simulink model "FourWheelSim_base"  (R2021b)
settings: Solver=ode4  StartTime=0.0  StopTime=100  FixedStep=0.001  EnableMultiTasking=on
values from neighbouring files (symbols this model uses):
  a_f = [1.434106444513048,-3.490394354141787e-04,2.761516722659314,6.000050177239062e+04,2.990012596710455e+03,-1.736376596503330e-04,0.526021936511837]    [VehicleParams20_ver230707.m]
  a_r = a_f    [VehicleParams20_ver230707.m]
  afx_f = [1.736519934348130,-2.903281841026900e-04,2.651682004580759,7.000047010028531e+04,3.270011055825476e+03,-0.001252141095807,1.596836353939939]    [VehicleParams20_ver230707.m]
  afx_r = afx_f    [VehicleParams20_ver230707.m]
  agx_f = [0.230000000000000,2.936116597489246e+04,7.137436879966481e+03,0,0]    [VehicleParams20_ver230707.m]
  agx_r = agx_f    [VehicleParams20_ver230707.m]
  agy_f = [0.852564208514954,3.000069064154418e+04,2.070023877794581e+03,-5.089267464508360e-04,0.519364283925805]    [VehicleParams20_ver230707.m]
  agy_r = agy_f    [VehicleParams20_ver230707.m]
  b_f = [3.436650779629654,1.566044221042620e-05,0.028598122547093,3.408741969645286e+03,5.995144285148312e+03,-1.736376595720277e-04,0.526021936449385]    [VehicleParams20_ver230707.m]
  Brake_Factor = 0.66    [VehicleParams20_ver230707.m]
  Cd = Cd/(40/3.6)^2    (= 0.6885)    [VehicleParams20_ver230707.m]
  CLF = DFf/40/40    (= 0.06)    [VehicleParams20_ver230707.m]
  CLR = DFr/40/40    (= 0.065)    [VehicleParams20_ver230707.m]
  cPiston_Area_F = 2*pi*(0.0254/2)^2    (= 0.00101341495819)    [VehicleParams20_ver230707.m]
  cPiston_Area_R = 2*pi*(0.0254/2)^2    (= 0.00101341495819)    [VehicleParams20_ver230707.m]
  delta = 15.5    [VehicleParams20_ver230707.m]
  df = 1.225    [VehicleParams20_ver230707.m]
  dr = 1.225    [VehicleParams20_ver230707.m]
  eff_Radius_F = (180/2-13.5)/1000    (= 0.0765)    [VehicleParams20_ver230707.m]
  eff_Radius_R = (180/2-13.5)/1000    (= 0.0765)    [VehicleParams20_ver230707.m]
  Fd = 60*2    (= 120)    [VehicleParams20_ver230707.m]
  Frtoe = 0    [VehicleParams20_ver230707.m]
  gear_f = 13.75    [VehicleParams20_ver230707.m]
  gear_r = 13.75    [VehicleParams20_ver230707.m]
  hg = 0.28    [VehicleParams20_ver230707.m]
  HV_voltage = 600    [VehicleParams20_ver230707.m]
  I = 112    [VehicleParams20_ver230707.m]
  ini_v = ini_speed/3.6    (= 10.4166666667)    [VehicleParams20_ver230707.m]
  Kframe = 5.94*10^6    (= 5940000)    [VehicleParams20_ver230707.m]
  kk_f = 2800*180/pi    (= 160428.182637)    [VehicleParams20_ver230707.m]
  kk_r = 4200*180/pi    (= 240642.273955)    [VehicleParams20_ver230707.m]
  krfr = 0.5    [VehicleParams20_ver230707.m]
  l = 1.530    (= 1.53)    [VehicleParams20_ver230707.m]
  lf = l*(1-WBf)    (= 0.7956)    [VehicleParams20_ver230707.m]
  lr = l*WBf    (= 0.7344)    [VehicleParams20_ver230707.m]
  M = 200+60    (= 260)    [VehicleParams20_ver230707.m]
  mu_tire_F = 0.587-0.587+0.55    (= 0.55)    [VehicleParams20_ver230707.m]
  mu_tire_R = 0.587-0.587+0.55    (= 0.55)    [VehicleParams20_ver230707.m]
  Mwf = Iwf/Rwf/Rwf    (= 3.82716814816)    [VehicleParams20_ver230707.m]
  Mwr = Iwr/Rwr/Rwr    (= 3.82716814816)    [VehicleParams20_ver230707.m]
  rcf = 0.000    (= 0)    [VehicleParams20_ver230707.m]
  rch = rcf*WBf+rcr*(1-WBf)    (= 0)    [VehicleParams20_ver230707.m]
  rcr = 0.000    (= 0)    [VehicleParams20_ver230707.m]
  Reartoe = -2    [VehicleParams20_ver230707.m]
  Rr_toe = Reartoe*pi/180    (= -0.0349065850399)    [VehicleParams20_ver230707.m]
  Rwf = 18*(25.4/1000)/2    (= 0.2286)    [VehicleParams20_ver230707.m]
  Rwr = 18*(25.4/1000)/2    (= 0.2286)    [VehicleParams20_ver230707.m]
  T_TireF = TireL_f/V    (= 0.036760000032)    [VehicleParams20_ver230707.m]
  T_TireR = TireL_r/V    (= 0.036760000032)    [VehicleParams20_ver230707.m]
  tspeed = 37.5    [VehicleParams20_ver230707.m]
  WBf = 0.48    [VehicleParams20_ver230707.m]
  zc_f = castrail_Fr/1000    (= 0)    [VehicleParams20_ver230707.m]
  zc_r = castrail_Rr/1000    (= 0)    [VehicleParams20_ver230707.m]
libraries: simulink x25, dspstat3 x1
(part 2 of 4)

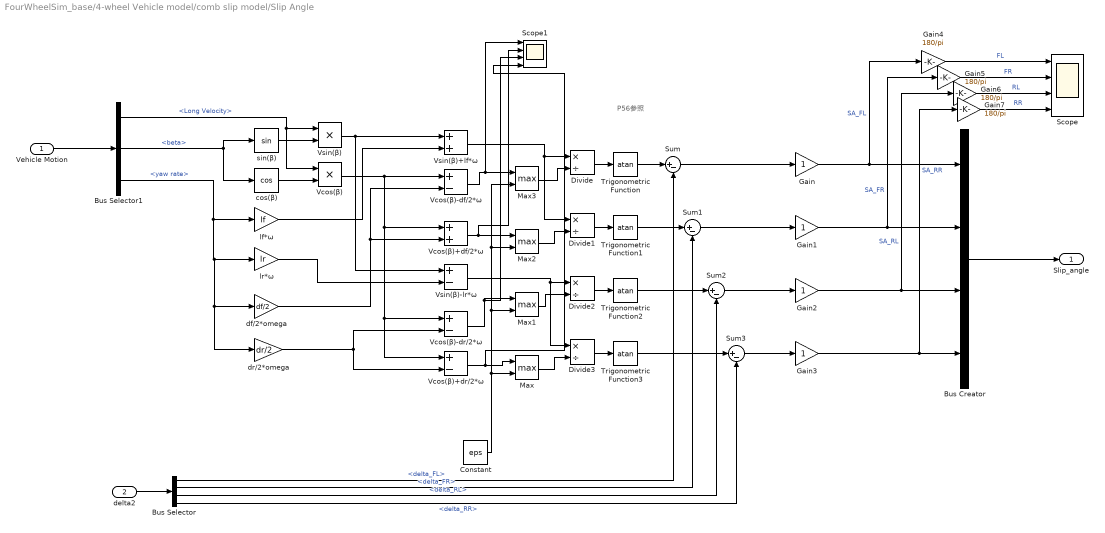
== system FourWheelSim_base/4-wheel Vehicle model/comb slip model/Slip Angle ==
  note: P56参照
  Vehicle Motion : Inport
  delta2 : Inport  Port=2
  Bus Creator : BusCreator  Inputs=4
  Bus Selector : BusSelector  OutputSignals=delta_FL,delta_FR,delta_RL,delta_RR
  Bus Selector1 : BusSelector  OutputSignals=Long Velocity,beta,yaw rate
  Constant : Constant  Value=eps
  Divide{,1..3} (4 alike) : Product  Inputs=*/
  Gain{,1..3} (4 alike) : Gain
  Gain{4..7} (4 alike) : Gain  Gain=180/pi
  Max{,1..3} (4 alike) : MinMax  Function=max  Inputs=2
  Scope : Scope  NumInputPorts=4
  Scope1 : Scope  NumInputPorts=4
  Sum{,1..3} (4 alike) : Sum  Inputs=|+-
  Trigonometric Function{,1..3} (4 alike) : Trigonometry  Operator=atan
  Vcos(β) : Product  Inputs=**
  Vcos(β)+df/2*ω : Sum
  Vcos(β)+dr/2*ω : Sum  Inputs=+-
  Vcos(β)-df/2*ω : Sum  Inputs=+-
  Vcos(β)-dr/2*ω : Sum  Inputs=+-
  Vsin(β) : Product  Inputs=**
  Vsin(β)+lf*ω : Sum
  Vsin(β)-lr*ω : Sum  Inputs=+-
  cos(β) : Trigonometry  Operator=cos
  df/2*omega : Gain  Gain=df/2
  dr/2*omega : Gain  Gain=dr/2
  lf*ω : Gain  Gain=lf
  lr*ω : Gain  Gain=lr
  sin(β) : Trigonometry
  Slip_angle : Outport  VectorParamsAs1DForOutWhenUnconnected=off
  wires:
  Bus Selector1/2 -> sin(β)/1, cos(β)/1  "<beta>"
  Bus Selector1/3 -> dr/2*omega/1, df/2*omega/1, lr*ω/1, lf*ω/1  "<yaw rate>"
  sin(β)/1 -> Vsin(β)/2
  cos(β)/1 -> Vcos(β)/2
  Vsin(β)/1 -> Vsin(β)-lr*ω/1, Vsin(β)+lf*ω/1
  lf*ω/1 -> Vsin(β)+lf*ω/2
  df/2*omega/1 -> Vcos(β)+df/2*ω/2, Vcos(β)-df/2*ω/2
  Vsin(β)+lf*ω/1 -> Divide1/1, Divide/1
  lr*ω/1 -> Vsin(β)-lr*ω/2
  Vcos(β)/1 -> Vcos(β)+df/2*ω/1, Vcos(β)+dr/2*ω/1, Vcos(β)-dr/2*ω/1, Vcos(β)-df/2*ω/1
  dr/2*omega/1 -> Vcos(β)-dr/2*ω/2, Vcos(β)+dr/2*ω/2
  Vsin(β)-lr*ω/1 -> Divide3/1, Divide2/1
  Bus Selector/1 -> Sum/2  "<delta_FL>"
  Trigonometric Function/1 -> Sum/1
  Sum/1 -> Gain/1
  Bus Selector/2 -> Sum1/2  "<delta_FR>"
  Trigonometric Function1/1 -> Sum1/1
  Sum1/1 -> Gain1/1
  Bus Selector/3 -> Sum2/2  "<delta_RL>"
  Trigonometric Function2/1 -> Sum2/1
  Bus Selector/4 -> Sum3/2  "<delta_RR>"
  Trigonometric Function3/1 -> Sum3/1
  Sum3/1 -> Gain3/1
  Sum2/1 -> Gain2/1
  Gain/1 -> Gain4/1, Bus Creator/1  "SA_FL"
  Gain1/1 -> Gain5/1, Bus Creator/2  "SA_FR"
  Gain2/1 -> Bus Creator/3, Gain6/1  "SA_RL"
  Gain3/1 -> Gain7/1, Bus Creator/4  "SA_RR"
  Bus Selector1/1 -> Vsin(β)/1, Vcos(β)/1  "<Long Velocity>"
  Bus Creator/1 -> Slip_angle/1
  delta2/1 -> Bus Selector/1
  Vehicle Motion/1 -> Bus Selector1/1
  Divide3/1 -> Trigonometric Function3/1
  Divide2/1 -> Trigonometric Function2/1
  Divide1/1 -> Trigonometric Function1/1
  Divide/1 -> Trigonometric Function/1
  Constant/1 -> Max3/2, Max2/2, Max1/2, Max/2
  Vcos(β)+dr/2*ω/1 -> Scope1/4, Max/1
  Vcos(β)+df/2*ω/1 -> Scope1/2, Max2/1
  Vcos(β)-df/2*ω/1 -> Scope1/1, Max3/1
  Vcos(β)-dr/2*ω/1 -> Scope1/3, Max1/1
  Max3/1 -> Divide/2
  Max2/1 -> Divide1/2
  Max1/1 -> Divide2/2
  Max/1 -> Divide3/2
  Gain4/1 -> Scope/1  "FL"
  Gain5/1 -> Scope/2  "FR"
  Gain6/1 -> Scope/3  "RL"
  Gain7/1 -> Scope/4  "RR"

== system FourWheelSim_base/4-wheel Vehicle model/comb slip model/Slip rate calc ==
  VehicleSpeed : Inport
  Wheel Speed : Inport  Port=2
  Bus Creator : BusCreator  Inputs=4
  Bus Selector : BusSelector  OutputSignals=Wheel_Speed_FL,Wheel_Speed_FR,Wheel_Speed_RL,Wheel_Speed_RR
  Bus Selector1 : BusSelector  OutputSignals=Long Velocity
  SlipRateClc{,1..3} (4 alike) : Subsystem  ReferencedSubsystem=SlipRateClc
  "SlipRate " : Outport  VectorParamsAs1DForOutWhenUnconnected=off
  wires:
  SlipRateClc2/1 -> Bus Creator/3  "Sliprate_RL"
  SlipRateClc1/1 -> Bus Creator/2  "Sliprate_FR"
  SlipRateClc/1 -> Bus Creator/1  "Sliprate_FL"
  SlipRateClc3/1 -> Bus Creator/4  "Sliprate_RR"
  Bus Selector1/1 -> SlipRateClc3/2, SlipRateClc2/2, SlipRateClc1/2, SlipRateClc/2  "<Long Velocity>"
  Bus Creator/1 -> "SlipRate "/1
  Wheel Speed/1 -> Bus Selector/1
  Bus Selector/4 -> SlipRateClc3/1  "<Wheel_Speed_RR>"
  Bus Selector/2 -> SlipRateClc1/1  "<Wheel_Speed_FR>"
  Bus Selector/1 -> SlipRateClc/1  "<Wheel_Speed_FL>"
  VehicleSpeed/1 -> Bus Selector1/1
  Bus Selector/3 -> SlipRateClc2/1  "<Wheel_Speed_RL>"

== system FourWheelSim_base/4-wheel Vehicle model/comb slip model/Wheel speed calc ==
  note: Unit : m/s
  comb_Fx : Inport
  Torque : Inport  Port=2
  1/r : Gain  Gain=1/Rwf
  1/r1 : Gain  Gain=1/Rwf
  1/r2 : Gain  Gain=1/Rwr
  1/r3 : Gain  Gain=1/Rwr
  Bus Creator : BusCreator  Inputs=4
  Bus Selector : BusSelector  OutputSignals=FL,RL,FR,RR
  Bus Selector1 : BusSelector  OutputSignals=Fx.Fx_FL,Fx.Fx_RL,Fx.Fx_FR,Fx.Fx_RR
  Gain17 : Gain  Gain=1/Mwf
  Gain18 : Gain  Gain=1/Mwf
  Gain19 : Gain  Gain=1/Mwr
  Gain20 : Gain  Gain=1/Mwr
  Scope : Scope  NumInputPorts=4
  Scope1 : Scope  NumInputPorts=4
  Scope2 : Scope  NumInputPorts=4
  Sum{2..3,13..14} (4 alike) : Sum  Inputs=|+-
  wheel speed F_in : Integrator  InitialCondition=ini_v  LimitOutput=on  LowerSaturationLimit=0
  wheel speed F_out : Integrator  InitialCondition=ini_v  LimitOutput=on  LowerSaturationLimit=0
  wheel speed R_in : Integrator  InitialCondition=ini_v  LimitOutput=on  LowerSaturationLimit=0
  wheel speed R_out : Integrator  InitialCondition=ini_v  LimitOutput=on  LowerSaturationLimit=0
  Wheel Speed : Outport  VectorParamsAs1DForOutWhenUnconnected=off
  wires:
  wheel speed R_out/1 -> Scope/4, Bus Creator/4  "Wheel_Speed_RR"
  Sum2/1 -> Gain18/1
  Sum14/1 -> Gain19/1
  wheel speed F_in/1 -> Scope/1, Bus Creator/1  "Wheel_Speed_FL"
  Gain19/1 -> wheel speed R_in/1
  Gain18/1 -> wheel speed F_out/1
  Sum3/1 -> Gain17/1
  Gain17/1 -> wheel speed F_in/1
  Sum13/1 -> Gain20/1
  Gain20/1 -> wheel speed R_out/1
  wheel speed F_out/1 -> Scope/2, Bus Creator/2  "Wheel_Speed_RL"
  wheel speed R_in/1 -> Scope/3, Bus Creator/3  "Wheel_Speed_FR"
  Bus Creator/1 -> Wheel Speed/1
  Torque/1 -> Bus Selector/1
  Bus Selector/1 -> Scope1/1, 1/r/1  "<FL>"
  Bus Selector/2 -> Scope1/2, 1/r2/1  "<RL>"
  Bus Selector/3 -> Scope1/3, 1/r1/1  "<FR>"
  Bus Selector/4 -> 1/r3/1, Scope1/4  "<RR>"
  comb_Fx/1 -> Bus Selector1/1
  Bus Selector1/1 -> Scope2/1, Sum3/2  "<Fx_FL>"
  Bus Selector1/2 -> Scope2/2, Sum2/2  "<Fx_RL>"
  Bus Selector1/3 -> Scope2/3, Sum14/2  "<Fx_FR>"
  Bus Selector1/4 -> Scope2/4, Sum13/2  "<Fx_RR>"
  1/r/1 -> Sum3/1
  1/r1/1 -> Sum14/1
  1/r2/1 -> Sum2/1
  1/r3/1 -> Sum13/1

== system FourWheelSim_base/4-wheel Vehicle model/comb slip model/comb Fx calc ==
  tire status : Inport
  Bus Creator : BusCreator  Inputs=4
  Bus Selector : BusSelector  OutputSignals=load.Load_FL,Slip angle.SA_FL,Slip rate.Sliprate_FL
  Bus Selector1 : BusSelector  OutputSignals=load.Load_FR,Slip angle.SA_FR,Slip rate.Sliprate_FR
  Bus Selector2 : BusSelector  OutputSignals=load.Load_RL,Slip angle.SA_RL,Slip rate.Sliprate_RL
  Bus Selector3 : BusSelector  OutputSignals=load.Load_RR,Slip angle.SA_RR,Slip rate.Sliprate_RR
  Force_Fin_comb_FX : Subsystem
  Force_Fout_comb_FX : Subsystem
  Force_Rin_comb_FX : Subsystem
  Force_Rout_comb1_FX : Subsystem
  Fx : Outport  VectorParamsAs1DForOutWhenUnconnected=off
  wires:
  Bus Creator/1 -> Fx/1
  Force_Fout_comb_FX/1(Force_Fout) -> Bus Creator/2  "Fx_FR"
  Force_Fin_comb_FX/1(Force_Fin) -> Bus Creator/1  "Fx_FL"
  Force_Rin_comb_FX/1(Force_Rin) -> Bus Creator/3  "Fx_RL"
  Force_Rout_comb1_FX/1(Force_Rin) -> Bus Creator/4  "Fx_RR"
  tire status/1 -> Bus Selector3/1, Bus Selector2/1, Bus Selector/1, Bus Selector1/1
  Bus Selector/1 -> Force_Fin_comb_FX/1(W_Fin)  "<Load_FL>"
  Bus Selector/2 -> Force_Fin_comb_FX/2(beta_Fin)  "<SA_FL>"
  Bus Selector/3 -> Force_Fin_comb_FX/3(slip rate)  "<Sliprate_FL>"
  Bus Selector1/1 -> Force_Fout_comb_FX/1(W_Fout)  "<Load_FR>"
  Bus Selector1/2 -> Force_Fout_comb_FX/2(beta_Fout)  "<SA_FR>"
  Bus Selector1/3 -> Force_Fout_comb_FX/3(slip rate)  "<Sliprate_FR>"
  Bus Selector2/1 -> Force_Rin_comb_FX/1(W_Rin)  "<Load_RL>"
  Bus Selector2/2 -> Force_Rin_comb_FX/2(beta_Rin)  "<SA_RL>"
  Bus Selector2/3 -> Force_Rin_comb_FX/3(slip rate)  "<Sliprate_RL>"
  Bus Selector3/1 -> Force_Rout_comb1_FX/1(W_Rout)  "<Load_RR>"
  Bus Selector3/2 -> Force_Rout_comb1_FX/2(beta_Rout)  "<SA_RR>"
  Bus Selector3/3 -> Force_Rout_comb1_FX/3(slip rate)  "<Sliprate_RR>"

== system FourWheelSim_base/4-wheel Vehicle model/comb slip model/comb Fy calc ==
  tire status : Inport
  Bus Creator : BusCreator  Inputs=4
  Bus Selector : BusSelector  OutputSignals=load.Load_FL,Slip angle.SA_FL,Slip rate.Sliprate_FL
  Bus Selector1 : BusSelector  OutputSignals=load.Load_FR,Slip angle.SA_FR,Slip rate.Sliprate_FR
  Bus Selector2 : BusSelector  OutputSignals=load.Load_RL,Slip angle.SA_RL,Slip rate.Sliprate_RL
  Bus Selector3 : BusSelector  OutputSignals=load.Load_RR,Slip angle.SA_RR,Slip rate.Sliprate_RR
  Force_Fin_comb_FY : Subsystem
  Force_Fout_comb_FY : Subsystem
  Force_Rin_comb_FY : Subsystem
  Force_Rout_comb_FY : Subsystem
  Fy : Outport  VectorParamsAs1DForOutWhenUnconnected=off
  wires:
  Bus Creator/1 -> Fy/1
  Force_Fout_comb_FY/1(Force_Fout) -> Bus Creator/2  "Fy_FR"
  Force_Fin_comb_FY/1(Force_Fin) -> Bus Creator/1  "Fy_FL"
  Force_Rin_comb_FY/1(Force_Rin) -> Bus Creator/3  "Fy_RL"
  Force_Rout_comb_FY/1(Force_Rout) -> Bus Creator/4  "Fy_RR"
  Bus Selector/3 -> Force_Fin_comb_FY/3(slip rate)  "<Sliprate_FL>"
  Bus Selector3/3 -> Force_Rout_comb_FY/3(slip rate)  "<Sliprate_RR>"
  Bus Selector2/1 -> Force_Rin_comb_FY/1(W_Fin)  "<Load_RL>"
  Bus Selector1/1 -> Force_Fout_comb_FY/1(W_Fin)  "<Load_FR>"
  Bus Selector1/2 -> Force_Fout_comb_FY/2(beta_Fin)  "<SA_FR>"
  tire status/1 -> Bus Selector3/1, Bus Selector2/1, Bus Selector/1, Bus Selector1/1
  Bus Selector1/3 -> Force_Fout_comb_FY/3(slip rate)  "<Sliprate_FR>"
  Bus Selector2/3 -> Force_Rin_comb_FY/3(slip rate)  "<Sliprate_RL>"
  Bus Selector2/2 -> Force_Rin_comb_FY/2(beta_Fin)  "<SA_RL>"
  Bus Selector/2 -> Force_Fin_comb_FY/2(beta_Fin)  "<SA_FL>"
  Bus Selector/1 -> Force_Fin_comb_FY/1(W_Fin)  "<Load_FL>"
  Bus Selector3/2 -> Force_Rout_comb_FY/2(beta_Fin)  "<SA_RR>"
  Bus Selector3/1 -> Force_Rout_comb_FY/1(W_Fin)  "<Load_RR>"

== system FourWheelSim_base/4-wheel Vehicle model/equation of motion /Beta Angle ==
  Lat Velo : Inport
  Long Velo : Inport  Port=2
  Atan : Trigonometry  Operator=atan
  Constant : Constant  Value=eps
  Divide : Product  Inputs=*/
  Max : MinMax  Function=max  Inputs=2
  Body Beta Angle : Outport  VectorParamsAs1DForOutWhenUnconnected=off
  tag scope: B=global
  wires:
  Lat Velo/1 -> Divide/1
  Max/1 -> Divide/2
  Divide/1 -> Atan/1
  Atan/1 -> [B], Body Beta Angle/1
  Long Velo/1 -> Max/1
  Constant/1 -> Max/2

== system FourWheelSim_base/4-wheel Vehicle model/equation of motion /GPS cordinate Clc ==
  Long Velo : Inport
  Lat Velo : Inport  Port=2
  YawAngle : Inport  Port=3
  Add : Sum  Inputs=+-
  Add1 : Sum
  Cos : Trigonometry  Operator=cos
  Cos1 : Trigonometry  Operator=cos
  Divide{,1..3} (4 alike) : Product  Inputs=**
  Integrator1 : Integrator
  Integrator2 : Integrator
  Sin : Trigonometry
  Sin1 : Trigonometry
  GPS East : Outport  VectorParamsAs1DForOutWhenUnconnected=off
  GPS North : Outport  Port=2  VectorParamsAs1DForOutWhenUnconnected=off
  wires:
  Long Velo/1 -> Divide1/1, Divide/1
  Divide/1 -> Add/1
  Add1/1 -> Integrator2/1
  Cos/1 -> Divide/2
  Integrator1/1 -> GPS East/1  "GPS East"
  Sin/1 -> Divide1/2
  Integrator2/1 -> GPS North/1  "GPS North"
  Sin1/1 -> Divide3/2
  Cos1/1 -> Divide2/2
  YawAngle/1 -> Cos/1, Cos1/1, Sin/1, Sin1/1
  Lat Velo/1 -> Divide3/1, Divide2/1
  Divide3/1 -> Add/2
  Add/1 -> Integrator1/1
  Divide1/1 -> Add1/1
  Divide2/1 -> Add1/2

== system FourWheelSim_base/4-wheel Vehicle model/equation of motion /Net Long Force ==
  Vehicle speed : Inport
  Long Force : Inport  Port=2
  Delay : Delay  DelayLength=1
  Gain16 : Gain  Gain=Cd
  Product : Product
  Rolling resistance : Constant  Value=Fd
  Sum1 : Sum  Inputs=|+-
  Sum3 : Sum  Inputs=|+-
  Net Long Force : Outport  VectorParamsAs1DForOutWhenUnconnected=off
  wires:
  Sum3/1 -> Sum1/1
  Long Force/1 -> Sum3/1
  Product/1 -> Gain16/1
  Rolling resistance/1 -> Sum3/2
  Gain16/1 -> Sum1/2  "Drag Force"
  Vehicle speed/1 -> Delay/1
  Sum1/1 -> Net Long Force/1
  Delay/1 -> Product/2, Product/1

== system FourWheelSim_base/4-wheel Vehicle model/equation of motion /Roll Clc ==
  note: ロール剛性を適当に0.0001にしてあるが
      | 本来の値が求められるなら変えたい
  Lat Acc : Inport
  Add : Sum  Inputs=+-
  Constant : Constant  Value=0.001
  Delay : Delay  DelayLength=1
  Divide : Product  Inputs=*/
  Gain : Gain  Gain=180/pi
  Roll rad : Gain  Gain=M*(hg-rch)*0.0001
  Scope : Scope
  RollRate : Outport  VectorParamsAs1DForOutWhenUnconnected=off
  RollAngle : Outport  Port=2  VectorParamsAs1DForOutWhenUnconnected=off
  wires:
  Delay/1 -> Add/2
  Constant/1 -> Divide/2
  Add/1 -> Divide/1
  Lat Acc/1 -> Roll rad/1
  Roll rad/1 -> Gain/1, RollAngle/1, Delay/1, Add/1  "RollAngle"
  Divide/1 -> RollRate/1  "RollRate"
  Gain/1 -> Scope/1

== system FourWheelSim_base/4-wheel Vehicle model/equation of motion /Yaw Clc ==
  Yaw Moment : Inport
  Moment/I : Gain  Gain=1/I
  yaw angle[rad] : Integrator
  yaw rate[rad/s] : Integrator
  yaw rate : Outport  VectorParamsAs1DForOutWhenUnconnected=off
  yaw angle : Outport  Port=2  VectorParamsAs1DForOutWhenUnconnected=off
  wires:
  yaw angle[rad]/1 -> yaw angle/1  "yaw angle"
  Moment/I/1 -> yaw rate[rad/s]/1
  yaw rate[rad/s]/1 -> yaw rate/1, yaw angle[rad]/1  "yaw rate"
  Yaw Moment/1 -> Moment/I/1

== system FourWheelSim_base/4-wheel Vehicle model/equation of motion /equation of motion ==
  Net Long Force : Inport
  Lat Force : Inport  Port=2
  yaw rate : Inport  Port=3
  Add : Sum
  Add1 : Sum  Inputs=-+
  Divide : Product  Inputs=**
  Divide1 : Product  Inputs=**
  Gain2 : Gain  Gain=1/3.6
  Integrator : Integrator  InitialConditionSource=external
  Integrator1 : Integrator
  Mass : Gain  Gain=1/M
  Mass2 : Gain  Gain=1/M
  Scope : Scope  NumInputPorts=2
  Scope1 : Scope  NumInputPorts=2
  Long Acc : Outport  VectorParamsAs1DForOutWhenUnconnected=off
  Long Velo : Outport  Port=2  VectorParamsAs1DForOutWhenUnconnected=off
  Lat Acc : Outport  Port=3  VectorParamsAs1DForOutWhenUnconnected=off
  Lat Velo : Outport  Port=4  VectorParamsAs1DForOutWhenUnconnected=off
  wires:
  Divide/1 -> Add/2  "vr"
  Add/1 -> Integrator/1
  Add1/1 -> Scope1/1, Integrator1/1
  Mass2/1 -> Add/1, Long Acc/1  "Fx/M"
  Divide1/1 -> Add1/1  "ur"
  Lat Force/1 -> Mass/1
  Net Long Force/1 -> Mass2/1
  Mass/1 -> Add1/2, Scope1/2, Lat Acc/1  "Fy/M"
  Integrator1/1 -> Divide/2, Scope/2, Lat Velo/1  "v"
  Integrator/1 -> Long Velo/1, Divide1/1, Scope/1  "u"
  yaw rate/1 -> Divide1/2, Divide/1
  [TargetSpeed] -> Gain2/1
  Gain2/1 -> Integrator/2

== system FourWheelSim_base/4-wheel Vehicle model/force direction change/Lat Force and Yaw Moment1 ==
  In1 : Inport
  Bus Selector : BusSelector  OutputSignals=Fx.Fx_FL,delta sincos.sin(deltaFL)
  Bus Selector1 : BusSelector  OutputSignals=Fy.Fy_FL,delta sincos.cos(deltaFL)
  Bus Selector2 : BusSelector  OutputSignals=Fx.Fx_FR,delta sincos.sin(deltaFR)
  Bus Selector3 : BusSelector  OutputSignals=Fy.Fy_FR,delta sincos.cos(deltaFR)
  Bus Selector4 : BusSelector  OutputSignals=Fx.Fx_RL,delta sincos.sin(deltaRL)
  Bus Selector5 : BusSelector  OutputSignals=Fy.Fy_RL,delta sincos.cos(deltaRL)
  Bus Selector6 : BusSelector  OutputSignals=Fx.Fx_RR,delta sincos.sin(deltaRR)
  Bus Selector7 : BusSelector  OutputSignals=Fy.Fy_RR,delta sincos.cos(deltaRR)
  FXsin(-Rr_Toe) : Product  Inputs=**
  FXsin(Rr_Toe) : Product  Inputs=**
  FXsin(delta) : Product  Inputs=**
  FXsin(delta)1 : Product  Inputs=**
  FYcos(-Rr_Toe) : Product  Inputs=**
  FYcos(Rr_Toe) : Product  Inputs=**
  FYcos(delta) : Product  Inputs=**
  FYcos(delta)1 : Product  Inputs=**
  Lat Force : Sum  Inputs=++++
  Sum{21..24} (4 alike) : Sum  Inputs=++|
  Yaw Moment : Sum  Inputs=++++
  lf : Gain  Gain=lf
  lf1 : Gain  Gain=lf
  lr : Gain  Gain=-lr
  lr1 : Gain  Gain=-lr
  Yaw_Moment : Outport  VectorParamsAs1DForOutWhenUnconnected=off
  Lat_Force : Outport  Port=2  VectorParamsAs1DForOutWhenUnconnected=off
  wires:
  Lat Force/1 -> Lat_Force/1
  Yaw Moment/1 -> Yaw_Moment/1
  FYcos(delta)/1 -> Sum21/2
  FYcos(Rr_Toe)/1 -> Sum24/2
  Sum23/1 -> Lat Force/3, lr/1
  FXsin(delta)/1 -> Sum21/1
  FXsin(-Rr_Toe)/1 -> Sum23/1
  Sum21/1 -> Lat Force/1, lf/1
  FXsin(delta)1/1 -> Sum22/1
  FYcos(delta)1/1 -> Sum22/2
  Sum22/1 -> Lat Force/2, lf1/1
  Sum24/1 -> Lat Force/4, lr1/1
  FYcos(-Rr_Toe)/1 -> Sum23/2
  FXsin(Rr_Toe)/1 -> Sum24/1
  lf/1 -> Yaw Moment/4
  lf1/1 -> Yaw Moment/3
  lr/1 -> Yaw Moment/2
  lr1/1 -> Yaw Moment/1
  In1/1 -> Bus Selector7/1, Bus Selector6/1, Bus Selector5/1, Bus Selector4/1, Bus Selector3/1, Bus Selector2/1, Bus Selector1/1, Bus Selector/1
  Bus Selector/1 -> FXsin(delta)/1  "<Fx_FL>"
  Bus Selector/2 -> FXsin(delta)/2  "<sin(deltaFL)>"
  Bus Selector1/1 -> FYcos(delta)/1  "<Fy_FL>"
  Bus Selector1/2 -> FYcos(delta)/2  "<cos(deltaFL)>"
  Bus Selector2/1 -> FXsin(delta)1/1  "<Fx_FR>"
  Bus Selector2/2 -> FXsin(delta)1/2  "<sin(deltaFR)>"
  Bus Selector3/1 -> FYcos(delta)1/1  "<Fy_FR>"
  Bus Selector3/2 -> FYcos(delta)1/2  "<cos(deltaFR)>"
  Bus Selector4/1 -> FXsin(-Rr_Toe)/1  "<Fx_RL>"
  Bus Selector4/2 -> FXsin(-Rr_Toe)/2  "<sin(deltaRL)>"
  Bus Selector5/1 -> FYcos(-Rr_Toe)/1  "<Fy_RL>"
  Bus Selector5/2 -> FYcos(-Rr_Toe)/2  "<cos(deltaRL)>"
  Bus Selector6/1 -> FXsin(Rr_Toe)/1  "<Fx_RR>"
  Bus Selector6/2 -> FXsin(Rr_Toe)/2  "<sin(deltaRR)>"
  Bus Selector7/1 -> FYcos(Rr_Toe)/1  "<Fy_RR>"
  Bus Selector7/2 -> FYcos(Rr_Toe)/2  "<cos(deltaRR)>"

== system FourWheelSim_base/4-wheel Vehicle model/force direction change/Long Force and Vectoring Yaw Moment ==
  In1 : Inport
  Bus Selector : BusSelector  OutputSignals=Fx.Fx_FL,delta sincos.cos(deltaFL)
  Bus Selector1 : BusSelector  OutputSignals=Fy.Fy_FL,delta sincos.sin(deltaFL)
  Bus Selector2 : BusSelector  OutputSignals=Fx.Fx_FR,delta sincos.cos(deltaFR)
  Bus Selector3 : BusSelector  OutputSignals=Fy.Fy_FR,delta sincos.sin(deltaFR)
  Bus Selector4 : BusSelector  OutputSignals=Fx.Fx_RL,delta sincos.cos(deltaRL)
  Bus Selector5 : BusSelector  OutputSignals=Fy.Fy_RL,delta sincos.sin(deltaRL)
  Bus Selector6 : BusSelector  OutputSignals=Fx.Fx_RR,delta sincos.cos(deltaRL)
  Bus Selector7 : BusSelector  OutputSignals=Fy.Fy_RR,delta sincos.sin(deltaRR)
  FXcos(-Rr_Toe) : Product  Inputs=**
  "FXcos(Rr_Toe)1 " : Product  Inputs=**
  FXcos(delta) : Product  Inputs=**
  FXcos(delta)1 : Product  Inputs=**
  FYsin(-Rr_Toe) : Product  Inputs=**
  FYsin(Rr_Toe)1 : Product  Inputs=**
  FYsin(delta) : Product  Inputs=**
  FYsin(delta)1 : Product  Inputs=**
  Long Force : Sum  Inputs=++++
  Sum{17..20} (4 alike) : Sum  Inputs=|+-
  Vectoring Yaw Moment : Sum  Inputs=++++
  df/2 : Gain  Gain=-df/2
  df/2_1 : Gain  Gain=-dr/2
  df/2_2 : Gain  Gain=df/2
  df/2_3 : Gain  Gain=dr/2
  Long_Force : Outport  VectorParamsAs1DForOutWhenUnconnected=off
  Vectoring_Yaw_Moment : Outport  Port=2  VectorParamsAs1DForOutWhenUnconnected=off
  wires:
  df/2_3/1 -> Vectoring Yaw Moment/1
  df/2_1/1 -> Vectoring Yaw Moment/2
  Sum20/1 -> df/2_3/1, Long Force/4
  Sum19/1 -> df/2_1/1, Long Force/3
  FXcos(-Rr_Toe)/1 -> Sum19/1
  Sum18/1 -> df/2_2/1, Long Force/2
  "FXcos(Rr_Toe)1 "/1 -> Sum20/1
  FXcos(delta)/1 -> Sum17/1
  FYsin(delta)1/1 -> Sum18/2
  FYsin(delta)/1 -> Sum17/2
  FXcos(delta)1/1 -> Sum18/1
  FYsin(Rr_Toe)1/1 -> Sum20/2
  FYsin(-Rr_Toe)/1 -> Sum19/2
  Sum17/1 -> df/2/1, Long Force/1
  df/2_2/1 -> Vectoring Yaw Moment/3
  df/2/1 -> Vectoring Yaw Moment/4
  Long Force/1 -> Long_Force/1
  Vectoring Yaw Moment/1 -> Vectoring_Yaw_Moment/1
  Bus Selector/1 -> FXcos(delta)/1  "<Fx_FL>"
  Bus Selector/2 -> FXcos(delta)/2  "<cos(deltaFL)>"
  In1/1 -> Bus Selector7/1, Bus Selector6/1, Bus Selector5/1, Bus Selector4/1, Bus Selector3/1, Bus Selector2/1, Bus Selector1/1, Bus Selector/1
  Bus Selector1/1 -> FYsin(delta)/1  "<Fy_FL>"
  Bus Selector1/2 -> FYsin(delta)/2  "<sin(deltaFL)>"
  Bus Selector2/1 -> FXcos(delta)1/1  "<Fx_FR>"
  Bus Selector2/2 -> FXcos(delta)1/2  "<cos(deltaFR)>"
  Bus Selector3/1 -> FYsin(delta)1/1  "<Fy_FR>"
  Bus Selector3/2 -> FYsin(delta)1/2  "<sin(deltaFR)>"
  Bus Selector4/1 -> FXcos(-Rr_Toe)/1  "<Fx_RL>"
  Bus Selector4/2 -> FXcos(-Rr_Toe)/2  "<cos(deltaRL)>"
  Bus Selector5/1 -> FYsin(-Rr_Toe)/1  "<Fy_RL>"
  Bus Selector5/2 -> FYsin(-Rr_Toe)/2  "<sin(deltaRL)>"
  Bus Selector6/1 -> "FXcos(Rr_Toe)1 "/1  "<Fx_RR>"
  Bus Selector6/2 -> "FXcos(Rr_Toe)1 "/2  "<cos(deltaRL)>"
  Bus Selector7/1 -> FYsin(Rr_Toe)1/1  "<Fy_RR>"
  Bus Selector7/2 -> FYsin(Rr_Toe)1/2  "<sin(deltaRR)>"

== system FourWheelSim_base/4-wheel Vehicle model/force direction change/sincos culc ==
  delta : Inport
  Bus Creator : BusCreator  Inputs=8
  Bus Selector : BusSelector  OutputSignals=delta_FL,delta_FR,delta_RL,delta_RR
  Cos{,1..3} (4 alike) : Trigonometry  Operator=cos
  Sin{,1..3} (4 alike) : Trigonometry
  delta sincos : Outport  VectorParamsAs1DForOutWhenUnconnected=off
  wires:
  Bus Selector/2 -> Cos/1, Sin/1  "<delta_FR>"
  Bus Selector/4 -> Cos2/1, Sin2/1  "<delta_RR>"
  Sin/1 -> Bus Creator/3  "sin(deltaFR)"
  Cos/1 -> Bus Creator/4  "cos(deltaFR)"
  Sin1/1 -> Bus Creator/5  "sin(deltaRL)"
  Cos1/1 -> Bus Creator/6  "cos(deltaRL)"
  Sin2/1 -> Bus Creator/7  "sin(deltaRR)"
  Cos2/1 -> Bus Creator/8  "cos(deltaRR)"
  Bus Creator/1 -> delta sincos/1
  Sin3/1 -> Bus Creator/1  "sin(deltaFL)"
  Cos3/1 -> Bus Creator/2  "cos(deltaFL)"
  delta/1 -> Bus Selector/1
  Bus Selector/1 -> Cos3/1, Sin3/1  "<delta_FL>"
  Bus Selector/3 -> Cos1/1, Sin1/1  "<delta_RL>"

== system FourWheelSim_base/Driver/Pylon Touch/R ==
  Abs : Abs
  Bus Creator : BusCreator  Inputs=2
  Cos : Trigonometry  Operator=cos
  Gain2 : Gain  Gain=-1
  Gain3 : Gain  Gain=-1
  Product : Product
  Product1 : Product
  Sin : Trigonometry
  R : Outport
  wires:
  [R] -> Abs/1
  [B] -> Cos/1, Sin/1
  Gain2/1 -> Product/2
  Abs/1 -> Product1/1, Product/1
  Cos/1 -> Gain3/1
  Gain3/1 -> Product1/2
  Product/1 -> Bus Creator/1  "Rx"
  Sin/1 -> Gain2/1
  Bus Creator/1 -> R/1
  Product1/1 -> Bus Creator/2  "Ry"

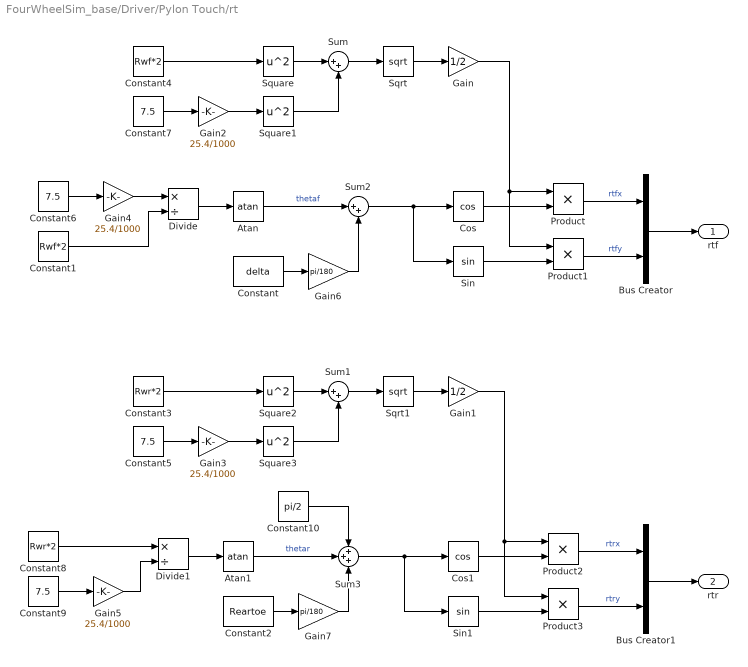
== system FourWheelSim_base/Driver/Pylon Touch/rt ==
  Atan : Trigonometry  Operator=atan
  Atan1 : Trigonometry  Operator=atan
  Bus Creator : BusCreator  Inputs=2
  Bus Creator1 : BusCreator  Inputs=2
  Constant : Constant  Value=delta
  Constant1 : Constant  Value=Rwf*2
  Constant10 : Constant  Value=pi/2
  Constant2 : Constant  Value=Reartoe
  Constant3 : Constant  Value=Rwr*2
  Constant4 : Constant  Value=Rwf*2
  Constant{5..7,9} (4 alike) : Constant  Value=7.5
  Constant8 : Constant  Value=Rwr*2
  Cos : Trigonometry  Operator=cos
  Cos1 : Trigonometry  Operator=cos
  Divide : Product  Inputs=*/
  Divide1 : Product  Inputs=*/
  Gain : Gain  Gain=1/2
  Gain1 : Gain  Gain=1/2
  Gain{2..5} (4 alike) : Gain  Gain=25.4/1000
  Gain6 : Gain  Gain=pi/180
  Gain7 : Gain  Gain=pi/180
  Product{,1..3} (4 alike) : Product
  Sin : Trigonometry
  Sin1 : Trigonometry
  Sqrt : Sqrt  SaturateOnIntegerOverflow=on
  Sqrt1 : Sqrt  SaturateOnIntegerOverflow=on
  Square{,1..3} (4 alike) : Math  Operator=square  SaturateOnIntegerOverflow=on
  Sum : Sum  Inputs=|++
  Sum1 : Sum  Inputs=|++
  Sum2 : Sum  Inputs=|++
  Sum3 : Sum  Inputs=+++
  rtf : Outport
  rtr : Outport  Port=2
  wires:
  Constant4/1 -> Square/1
  Gain2/1 -> Square1/1
  Square/1 -> Sum/1
  Square1/1 -> Sum/2
  Sum/1 -> Sqrt/1
  Sqrt/1 -> Gain/1
  Constant7/1 -> Gain2/1
  Constant5/1 -> Gain3/1
  Sqrt1/1 -> Gain1/1
  Sum1/1 -> Sqrt1/1
  Square3/1 -> Sum1/2
  Square2/1 -> Sum1/1
  Gain3/1 -> Square3/1
  Constant3/1 -> Square2/1
  Constant6/1 -> Gain4/1
  Gain4/1 -> Divide/1
  Constant1/1 -> Divide/2
  Divide/1 -> Atan/1
  Atan/1 -> Sum2/1  "thetaf"
  Constant/1 -> Gain6/1
  Sum2/1 -> Sin/1, Cos/1
  Cos/1 -> Product/2
  Sin/1 -> Product1/2
  Gain/1 -> Product1/1, Product/1
  Product/1 -> Bus Creator/1  "rtfx"
  Product1/1 -> Bus Creator/2  "rtfy"
  Constant2/1 -> Gain7/1
  Atan1/1 -> Sum3/2  "thetar"
  Divide1/1 -> Atan1/1
  Constant8/1 -> Divide1/1
  Gain5/1 -> Divide1/2
  Constant9/1 -> Gain5/1
  Constant10/1 -> Sum3/1
  Product3/1 -> Bus Creator1/2  "rtry"
  Product2/1 -> Bus Creator1/1  "rtrx"
  Gain1/1 -> Product2/1, Product3/1
  Sin1/1 -> Product3/2
  Cos1/1 -> Product2/2
  Sum3/1 -> Sin1/1, Cos1/1
  Bus Creator/1 -> rtf/1
  Bus Creator1/1 -> rtr/1
  Gain6/1 -> Sum2/2
  Gain7/1 -> Sum3/3

== system FourWheelSim_base/Driver/Pylon Touch/rw ==
  Bus Creator : BusCreator  Inputs=2
  Bus Creator1 : BusCreator  Inputs=2
  Constant : Constant
  Constant1 : Constant  Value=df/2
  Constant2 : Constant  Value=WBf
  Constant3 : Constant  Value=dr/2
  Gain : Gain  Gain=l
  Gain1 : Gain  Gain=-l
  Sum : Sum  Inputs=|+-
  rwf : Outport
  rwr : Outport  Port=2
  wires:
  Sum/1 -> Gain/1
  Gain1/1 -> Bus Creator1/1  "rwrx"
  Constant2/1 -> Sum/2, Gain1/1
  Gain/1 -> Bus Creator/1  "rwfx"
  Constant3/1 -> Bus Creator1/2  "rwry"
  Constant/1 -> Sum/1
  Constant1/1 -> Bus Creator/2  "rwfy"
  Bus Creator/1 -> rwf/1
  Bus Creator1/1 -> rwr/1

== system FourWheelSim_base/TractiveSystem/AMK PowerUnit x4/All Power consumption ==
  Motor trq : Inport
  Wheel speed : Inport  Port=2
  Add : Sum  Inputs=++++
  Bus Creator1 : BusCreator  Inputs=2
  Bus Selector1 : BusSelector  OutputSignals=Motor trq.FR Torque,Wheel Speed.Wheel_Speed_FR
  Bus Selector2 : BusSelector  OutputSignals=Motor trq.RR Torque,Wheel Speed.Wheel_Speed_RR
  Bus Selector3 : BusSelector  OutputSignals=Motor trq.RL Torque,Wheel Speed.Wheel_Speed_RL
  Bus Selector4 : BusSelector  OutputSignals=Motor trq.FL Torque,Wheel Speed.Wheel_Speed_FL
  Gain4 : Gain  Gain=gear_f*60/(2*Rwf*pi)
  Gain5 : Gain  Gain=gear_r*60/(2*Rwf*pi)
  Gain6 : Gain  Gain=gear_f*60/(2*Rwf*pi)
  Gain7 : Gain  Gain=gear_r*60/(2*Rwr*pi)
  Power Consumption clc{,1..3} (4 alike) : Subsystem  ReferencedSubsystem=Power_Consumption_clc
  All Power consumption [W] : Outport
  wires:
  Bus Selector1/1 -> Power Consumption clc/1  "<FR Torque>"
  Power Consumption clc2/1 -> Add/3
  Bus Selector1/2 -> Gain4/1  "<Wheel_Speed_FR>"
  Power Consumption clc/1 -> Add/1
  Gain7/1 -> Power Consumption clc2/2
  Power Consumption clc1/1 -> Add/2
  Power Consumption clc3/1 -> Add/4
  Bus Creator1/1 -> Bus Selector4/1, Bus Selector3/1, Bus Selector2/1, Bus Selector1/1
  Gain6/1 -> Power Consumption clc3/2
  Wheel speed/1 -> Bus Creator1/1
  Gain4/1 -> Power Consumption clc/2
  Gain5/1 -> Power Consumption clc1/2
  Add/1 -> All Power consumption [W]/1
  Motor trq/1 -> Bus Creator1/2
  Bus Selector2/2 -> Gain5/1  "<Wheel_Speed_RR>"
  Bus Selector2/1 -> Power Consumption clc1/1  "<RR Torque>"
  Bus Selector3/2 -> Gain7/1  "<Wheel_Speed_RL>"
  Bus Selector3/1 -> Power Consumption clc2/1  "<RL Torque>"
  Bus Selector4/2 -> Gain6/1  "<Wheel_Speed_FL>"
  Bus Selector4/1 -> Power Consumption clc3/1  "<FL Torque>"

== system FourWheelSim_base/TractiveSystem/AMK PowerUnit x4/CAN from Inv ==
  In1 : Inport
  In2 : Inport  Port=2
  In3 : Inport  Port=3
  In4 : Inport  Port=4
  In5 : Inport  Port=5
  In6 : Inport  Port=6
  In7 : Inport  Port=7
  In8 : Inport  Port=8
  In9 : Inport  Port=9
  In10 : Inport  Port=10
  In11 : Inport  Port=11
  In12 : Inport  Port=12
  Add : Sum  Inputs=++++
  Bus Creator2 : BusCreator  Inputs=12
  Bus Selector : BusSelector  OutputSignals=MC_13.MC1_Actual power value,MC_33.MC3_Actual power value,MC_23.MC2_Actual power value,MC_43.MC4_Actual power value
  Display : Display
  CAN from Inv : Outport  VectorParamsAs1DForOutWhenUnconnected=off
  wires:
  In4/1 -> Bus Creator2/4  "MC_31"
  In8/1 -> Bus Creator2/8  "MC_22"
  In2/1 -> Bus Creator2/2  "MC_12"
  In3/1 -> Bus Creator2/3  "MC_13"
  Bus Creator2/1 -> Bus Selector/1, CAN from Inv/1
  In1/1 -> Bus Creator2/1  "MC_11"
  In10/1 -> Bus Creator2/10  "MC_41"
  In11/1 -> Bus Creator2/11  "MC_42"
  In12/1 -> Bus Creator2/12  "MC_43"
  In6/1 -> Bus Creator2/6  "MC_33"
  In9/1 -> Bus Creator2/9  "MC_23"
  In5/1 -> Bus Creator2/5  "MC_32"
  In7/1 -> Bus Creator2/7  "MC_21"
  Bus Selector/1 -> Add/1  "<MC1_Actual power value>"
  Bus Selector/2 -> Add/2  "<MC3_Actual power value>"
  Bus Selector/3 -> Add/3  "<MC2_Actual power value>"
  Bus Selector/4 -> Add/4  "<MC4_Actual power value>"
  Add/1 -> Display/1

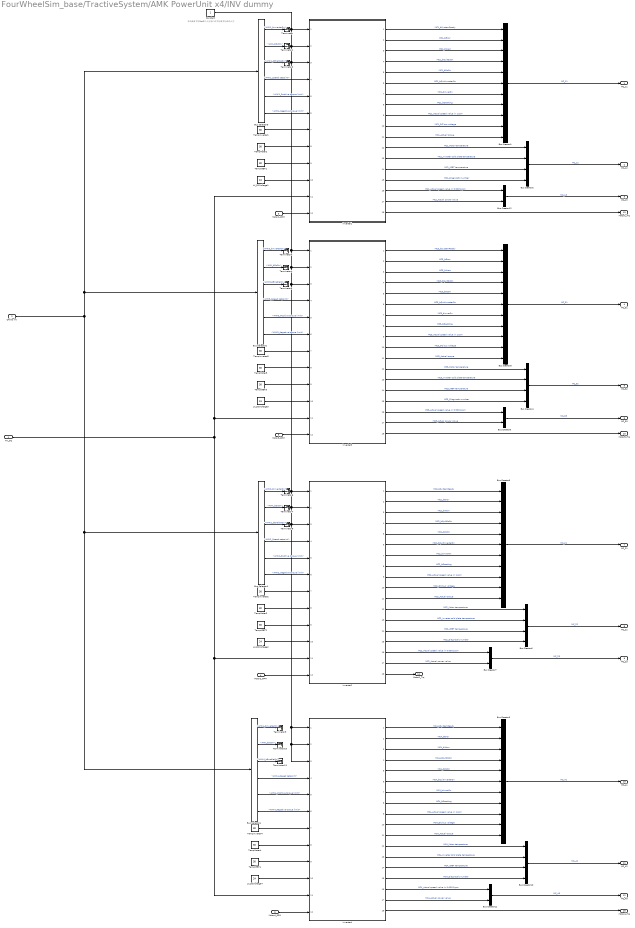
== system FourWheelSim_base/TractiveSystem/AMK PowerUnit x4/INV dummy ==
  note: そのままではRtoDに入らないのでだますための入力
  HV_DC : Inport
  CAN to Inv : Inport  Port=2
  Motor1_RPM : Inport  Port=3
  Motor2_RPM : Inport  Port=4
  Motor3_RPM : Inport  Port=5
  Motor4_RPM : Inport  Port=6
  Bus Creator{1,3,8..9} (4 alike) : BusCreator  Inputs=11
  Bus Creator{2,4,6,10} (4 alike) : BusCreator  Inputs=4
  Bus Creator{5,7,11..12} (4 alike) : BusCreator  Inputs=2
  Bus Selector1 : BusSelector  OutputSignals=AMK_21.AMK2_bInverterOn,AMK_21.AMK_bDcOn,AMK_21.AMK2_bEnableOn,AMK_21.AMK2_Speed setpoint,AMK_21.AMK2_Positive torque limit,AMK_21.AMK2_Negative torque limit
  Bus Selector2 : BusSelector  OutputSignals=AMK_31.AMK3_bInverterOn,AMK_31.AMK_bDcOn,AMK_31.AMK3_bEnableOn,AMK_31.AMK3_Speed setpoint,AMK_31.AMK3_Positive torque limit,AMK_31.AMK3_Negative torque limit
  Bus Selector3 : BusSelector  OutputSignals=AMK_11.AMK1_bInverterOn,AMK_11.AMK_bDcOn,AMK_11.AMK1_bEnableOn,AMK_11.AMK1_Speed setpoint,AMK_11.AMK1_Positive torque limit,AMK_11.AMK1_Negative torque limit
  Bus Selector4 : BusSelector  OutputSignals=AMK_41.AMK4_bInverterOn,AMK_41.AMK_bDcOn,AMK_41.AMK4_bEnableOn,AMK_41.AMK4_Speed setpoint,AMK_41.AMK4_Positive torque limit,AMK_41.AMK4_Negative torque limit
  Constant : Constant
  Inverter{1..4} (4 alike) : Subsystem  ReferencedSubsystem=PowerUnit_AMK
  LV_DCVoltage{1..4} (4 alike) : Constant  Value=24
  TempIGBT{1..4} (4 alike) : Constant  Value=30
  "TempInverter1 " : Constant  Value=30
  TempInverter2 : Constant  Value=30
  TempInverter3 : Constant  Value=30
  TempInverter4 : Constant  Value=30
  TempMoter{1..4} (4 alike) : Constant  Value=30
  Terminator{,1..11} (12 alike) : Terminator
  MC_11 : Outport  VectorParamsAs1DForOutWhenUnconnected=off
  MC_12 : Outport  Port=2  VectorParamsAs1DForOutWhenUnconnected=off
  MC_13 : Outport  Port=3  VectorParamsAs1DForOutWhenUnconnected=off
  MC_31 : Outport  Port=4  VectorParamsAs1DForOutWhenUnconnected=off
  MC_32 : Outport  Port=5  VectorParamsAs1DForOutWhenUnconnected=off
  MC_33 : Outport  Port=6  VectorParamsAs1DForOutWhenUnconnected=off
  MC_21 : Outport  Port=7  VectorParamsAs1DForOutWhenUnconnected=off
  MC_22 : Outport  Port=8  VectorParamsAs1DForOutWhenUnconnected=off
  MC_23 : Outport  Port=9  VectorParamsAs1DForOutWhenUnconnected=off
  MC_41 : Outport  Port=10  VectorParamsAs1DForOutWhenUnconnected=off
  MC_42 : Outport  Port=11  VectorParamsAs1DForOutWhenUnconnected=off
  MC_43 : Outport  Port=12  VectorParamsAs1DForOutWhenUnconnected=off
  Motor1_Trq : Outport  Port=13  VectorParamsAs1DForOutWhenUnconnected=off
  Motor2_Trq : Outport  Port=14  VectorParamsAs1DForOutWhenUnconnected=off
  Motor3_Trq : Outport  Port=15  VectorParamsAs1DForOutWhenUnconnected=off
  Motor4_Trq : Outport  Port=16  VectorParamsAs1DForOutWhenUnconnected=off
  wires:
  TempMoter1/1 -> Inverter1/8
  TempIGBT1/1 -> Inverter1/9
  LV_DCVoltage1/1 -> Inverter1/10
  "TempInverter1 "/1 -> Inverter1/7
  Bus Creator4/1 -> MC_32/1  "MC_32"
  HV_DC/1 -> Inverter4/11, Inverter2/11, Inverter3/11, Inverter1/11
  Bus Selector3/6 -> Inverter1/6  "<AMK1_Negative torque limit>"
  CAN to Inv/1 -> Bus Selector4/1, Bus Selector1/1, Bus Selector2/1, Bus Selector3/1
  Bus Selector3/5 -> Inverter1/5  "<AMK1_Positive torque limit>"
  Bus Creator5/1 -> MC_33/1  "MC_33"
  Bus Creator3/1 -> MC_31/1  "MC_31"
  Bus Selector3/4 -> Inverter1/4  "<AMK1_Speed setpoint>"
  Inverter3/1 -> Bus Creator3/1  "MC3_bSystemReady"
  Inverter3/2 -> Bus Creator3/2  "MC3_bError"
  Inverter3/3 -> Bus Creator3/3  "MC3_bWarn"
  Inverter3/4 -> Bus Creator3/4  "MC3_bQuitDcOn"
  Inverter3/5 -> Bus Creator3/5  "MC3_bDcOn"
  Inverter3/6 -> Bus Creator3/6  "MC3_bQuitInverterOn"
  Inverter3/7 -> Bus Creator3/7  "MC3_bInverOn"
  Inverter3/8 -> Bus Creator3/8  "MC3_bDerating"
  Inverter3/9 -> Bus Creator3/9  "MC3_Actual speed value in 1/rpm"
  Inverter3/10 -> Bus Creator3/10  "MC3_DC bus voltage"
  Inverter3/11 -> Bus Creator3/11  "MC3_Actual torque"
  Inverter3/12 -> Bus Creator4/1  "MC3_Motor temperature"
  Inverter3/13 -> Bus Creator4/2  "MC3_Inverter cold plate temperature"
  Inverter3/14 -> Bus Creator4/3  "MC3_IGBT temperature"
  Inverter3/15 -> Bus Creator4/4  "MC3_Diagnostic number"
  Inverter3/16 -> Bus Creator5/1  "MC3_Actual speed value in 0;0001/rpm"
  Inverter3/17 -> Bus Creator5/2  "MC3_Actual power value"
  TempMoter2/1 -> Inverter2/8
  TempIGBT2/1 -> Inverter2/9
  LV_DCVoltage2/1 -> Inverter2/10
  TempInverter2/1 -> Inverter2/7
  Bus Creator10/1 -> MC_42/1  "MC_42"
  Bus Creator11/1 -> MC_43/1  "MC_43"
  Bus Creator9/1 -> MC_41/1  "MC_41"
  Inverter4/1 -> Bus Creator9/1  "MC4_bSystemReady"
  Inverter4/2 -> Bus Creator9/2  "MC4_bError"
  Inverter4/3 -> Bus Creator9/3  "MC4_bWarn"
  Inverter4/4 -> Bus Creator9/4  "MC4_bQuitDcOn"
  Inverter4/5 -> Bus Creator9/5  "MC4_bDcOn"
  Inverter4/6 -> Bus Creator9/6  "MC4_bQuitInverterOn"
  Inverter4/7 -> Bus Creator9/7  "MC4_bInverOn"
  Inverter4/8 -> Bus Creator9/8  "MC4_bDerating"
  Inverter4/9 -> Bus Creator9/9  "MC4_Actual speed value in 1/rpm"
  Inverter4/10 -> Bus Creator9/10  "MC4_DC bus voltage"
  Inverter4/11 -> Bus Creator9/11  "MC4_Actual torque"
  Inverter4/12 -> Bus Creator10/1  "MC4_Motor temperature"
  Inverter4/13 -> Bus Creator10/2  "MC4_Inverter cold plate temperature"
  Inverter4/14 -> Bus Creator10/3  "MC4_IGBT temperature"
  Inverter4/15 -> Bus Creator10/4  "MC4_Diagnostic number"
  Inverter4/16 -> Bus Creator11/1  "MC4_Actual speed value in 0;0001/rpm"
  Inverter4/17 -> Bus Creator11/2  "MC4_Actual power value"
  Inverter2/18 -> Motor2_Trq/1
  Motor1_RPM/1 -> Inverter1/12
  Motor2_RPM/1 -> Inverter2/12
  Inverter3/18 -> Motor3_Trq/1
  Bus Selector2/4 -> Inverter3/4  "<AMK3_Speed setpoint>"
  Bus Selector2/5 -> Inverter3/5  "<AMK3_Positive torque limit>"
  Bus Selector2/6 -> Inverter3/6  "<AMK3_Negative torque limit>"
  TempIGBT3/1 -> Inverter3/9
  LV_DCVoltage3/1 -> Inverter3/10
  TempMoter3/1 -> Inverter3/8
  TempInverter3/1 -> Inverter3/7
  Inverter4/18 -> Motor4_Trq/1
  Bus Selector4/4 -> Inverter4/4  "<AMK4_Speed setpoint>"
  Bus Selector4/5 -> Inverter4/5  "<AMK4_Positive torque limit>"
  Bus Selector4/6 -> Inverter4/6  "<AMK4_Negative torque limit>"
  TempInverter4/1 -> Inverter4/7
  TempMoter4/1 -> Inverter4/8
  TempIGBT4/1 -> Inverter4/9
  LV_DCVoltage4/1 -> Inverter4/10
  Motor3_RPM/1 -> Inverter3/12
  Motor4_RPM/1 -> Inverter4/12
  Bus Selector1/4 -> Inverter2/4  "<AMK2_Speed setpoint>"
  Bus Selector1/5 -> Inverter2/5  "<AMK2_Positive torque limit>"
  Bus Selector1/6 -> Inverter2/6  "<AMK2_Negative torque limit>"
  Inverter1/14 -> Bus Creator2/3  "MC1_IGBT temperature"
  Inverter1/9 -> Bus Creator1/9  "MC1_Actual speed value in 1/rpm"
  Inverter1/5 -> Bus Creator1/5  "MC1_bDcOn"
  Inverter1/17 -> Bus Creator12/2  "MC1_Actual power value"
  Inverter1/2 -> Bus Creator1/2  "MC1_bError"
  Inverter1/3 -> Bus Creator1/3  "MC1_bWarn"
  Inverter1/1 -> Bus Creator1/1  "MC1_bSystemReady"
  Inverter1/13 -> Bus Creator2/2  "MC1_Inverter cold plate temperature"
  Inverter1/16 -> Bus Creator12/1  "MC1_Actual speed value in 0;0001/rpm"
  Bus Creator12/1 -> MC_13/1  "MC_13"
  Inverter1/12 -> Bus Creator2/1  "MC1_Motor temperature"
  Inverter1/8 -> Bus Creator1/8  "MC1_bDerating"
  Bus Creator2/1 -> MC_12/1  "MC_12"
  Inverter1/7 -> Bus Creator1/7  "MC1_bInverOn"
  Inverter1/10 -> Bus Creator1/10  "MC1_DC bus voltage"
  Inverter1/15 -> Bus Creator2/4  "MC1_Diagnostic number"
  Inverter1/11 -> Bus Creator1/11  "MC1_Actual torque"
  Bus Creator1/1 -> MC_11/1  "MC_11"
  Inverter1/4 -> Bus Creator1/4  "MC1_bQuitDcOn"
  Inverter1/6 -> Bus Creator1/6  "MC1_bQuitInverterOn"
  Inverter1/18 -> Motor1_Trq/1
  Inverter2/17 -> Bus Creator7/2  "MC2_Actual power value"
  Inverter2/16 -> Bus Creator7/1  "MC2_Actual speed value in 0;0001/rpm"
  Inverter2/15 -> Bus Creator6/4  "MC2_Diagnostic number"
  Inverter2/14 -> Bus Creator6/3  "MC2_IGBT temperature"
  Inverter2/13 -> Bus Creator6/2  "MC2_Inverter cold plate temperature"
  Inverter2/12 -> Bus Creator6/1  "MC2_Motor temperature"
  Inverter2/11 -> Bus Creator8/11  "MC2_Actual torque"
  Inverter2/10 -> Bus Creator8/10  "MC2_DC bus voltage"
  Inverter2/9 -> Bus Creator8/9  "MC2_Actual speed value in 1/rpm"
  Inverter2/8 -> Bus Creator8/8  "MC2_bDerating"
  Inverter2/7 -> Bus Creator8/7  "MC2_bInverOn"
  Inverter2/6 -> Bus Creator8/6  "MC2_bQuitInverterOn"
  Inverter2/5 -> Bus Creator8/5  "MC2_bDcOn"
  Inverter2/4 -> Bus Creator8/4  "MC2_bQuitDcOn"
  Inverter2/3 -> Bus Creator8/3  "MC2_bWarn"
  Inverter2/2 -> Bus Creator8/2  "MC2_bError"
  Inverter2/1 -> Bus Creator8/1  "MC2_bSystemReady"
  Bus Creator8/1 -> MC_21/1  "MC_21"
  Bus Creator7/1 -> MC_23/1  "MC_23"
  Bus Creator6/1 -> MC_22/1  "MC_22"
  Bus Selector3/1 -> Terminator/1  "<AMK1_bInverterOn>"
  Bus Selector3/2 -> Terminator1/1  "<AMK_bDcOn>"
  Bus Selector3/3 -> Terminator2/1  "<AMK1_bEnableOn>"
  Bus Selector2/3 -> Terminator5/1  "<AMK3_bEnableOn>"
  Bus Selector2/2 -> Terminator4/1  "<AMK_bDcOn>"
  Bus Selector2/1 -> Terminator3/1  "<AMK3_bInverterOn>"
  Bus Selector1/3 -> Terminator8/1  "<AMK2_bEnableOn>"
  Bus Selector1/2 -> Terminator7/1  "<AMK_bDcOn>"
  Bus Selector1/1 -> Terminator6/1  "<AMK2_bInverterOn>"
  Constant/1 -> Inverter3/3, Inverter4/3, Inverter4/2, Inverter4/1, Inverter2/3, Inverter2/2, Inverter2/1, Inverter3/2, Inverter3/1, Inverter1/3, Inverter1/2, Inverter1/1
  Bus Selector4/3 -> Terminator11/1  "<AMK4_bEnableOn>"
  Bus Selector4/2 -> Terminator10/1  "<AMK_bDcOn>"
  Bus Selector4/1 -> Terminator9/1  "<AMK4_bInverterOn>"

== system FourWheelSim_base/TractiveSystem/Sensors/NoiseGenerater ==
  note: SBGの説明書
      | Ellipse-N
      | Acc
      | Accuracy : 0.1m/s RMS
  X : Inport
  Add : Sum
  NoiseGenerater RMS0.1 : RandomNumber  Variance=0.01  SampleTime=0.001
  X+X' : Outport  VectorParamsAs1DForOutWhenUnconnected=off
  wires:
  NoiseGenerater RMS0.1/1 -> Add/2
  Add/1 -> X+X'/1  "X+X'"
  X/1 -> Add/1

== system FourWheelSim_base/TractiveSystem/Sensors/NoiseGenerater1 ==
  note: SBGの説明書
      | Ellipse-N
      | Acc
      | Accuracy : 0.1m/s RMS
  X : Inport
  Add : Sum
  NoiseGenerater RMS0.1 : RandomNumber  Variance=0.01  SampleTime=0.001
  X+X' : Outport  VectorParamsAs1DForOutWhenUnconnected=off
  wires:
  X/1 -> Add/1
  Add/1 -> X+X'/1  "X+X'"
  NoiseGenerater RMS0.1/1 -> Add/2

== system FourWheelSim_base/TractiveSystem/Sensors/NoiseGenerater2 ==
  note: SBGの説明書
      | Ellipse-N
      | Gyro
      | In run bias instability : 7deg/hr
      | 分散は適当
  X : Inport
  Add : Sum
  Random Number : RandomNumber  Mean=7/3600  Variance=0.001  SampleTime=0.001
  Scope : Scope  NumInputPorts=2
  X+X' : Outport  VectorParamsAs1DForOutWhenUnconnected=off
  wires:
  X/1 -> Scope/2, Add/1
  Add/1 -> Scope/1, X+X'/1  "X+X'"
  Random Number/1 -> Add/2

== system FourWheelSim_base/TractiveSystem/Sensors/NoiseGenerater3 ==
  note: SBGの説明書
      | Ellipse-N
      | Gyro
      | In run bias instability : 7deg/hr
      | 分散は適当
  X : Inport
  Add : Sum
  Random Number : RandomNumber  Mean=7/3600  Variance=0.001  SampleTime=0.001
  Scope : Scope
  X+X' : Outport  VectorParamsAs1DForOutWhenUnconnected=off
  wires:
  Random Number/1 -> Add/2
  Add/1 -> X+X'/1, Scope/1  "X+X'"
  X/1 -> Add/1

== system FourWheelSim_base/TractiveSystem/Sensors/NoiseGenerater4 ==
  note: SBGの説明書
      | Ellipse-N
      | Acc
      | In run bias instability : 3microg
      | 分散は適当
  X : Inport
  Add : Sum
  Random Number : RandomNumber  Mean=14*10^-6*9.8  Variance=0.0001  SampleTime=0.001
  Scope : Scope  NumInputPorts=2
  X+X' : Outport  VectorParamsAs1DForOutWhenUnconnected=off
  wires:
  Random Number/1 -> Add/2
  Add/1 -> X+X'/1, Scope/1  "X+X'"
  X/1 -> Add/1, Scope/2

== system FourWheelSim_base/TractiveSystem/Sensors/NoiseGenerater5 ==
  note: SBGの説明書
      | Ellipse-N
      | Acc
      | In run bias instability : 3microg
      | 分散は適当
  X : Inport
  Add : Sum
  Random Number : RandomNumber  Mean=14*10^-6*9.8  Variance=0.0001  SampleTime=0.001
  Scope : Scope  NumInputPorts=2
  X+X' : Outport  VectorParamsAs1DForOutWhenUnconnected=off
  wires:
  X/1 -> Scope/2, Add/1
  Add/1 -> Scope/1, X+X'/1  "X+X'"
  Random Number/1 -> Add/2

== system FourWheelSim_base/TractiveSystem/Sensors/differentialGPS ==
  X : Inport
  Add : Sum  Inputs=+-
  Constant6 : Constant  Value=0.001
  Delay19 : Delay  DelayLength=1
  Divide : Product  Inputs=*/
  X' : Outport  VectorParamsAs1DForOutWhenUnconnected=off
  wires:
  Add/1 -> Divide/1
  Constant6/1 -> Divide/2
  Divide/1 -> X'/1
  X/1 -> Delay19/1, Add/1
  Delay19/1 -> Add/2

== system FourWheelSim_base/TractiveSystem/Sensors/differentialGPS1 ==
  X : Inport
  Add : Sum  Inputs=+-
  Constant6 : Constant  Value=0.001
  Delay19 : Delay  DelayLength=1
  Divide : Product  Inputs=*/
  X' : Outport  VectorParamsAs1DForOutWhenUnconnected=off
  wires:
  Delay19/1 -> Add/2
  X/1 -> Add/1, Delay19/1
  Divide/1 -> X'/1
  Constant6/1 -> Divide/2
  Add/1 -> Divide/1

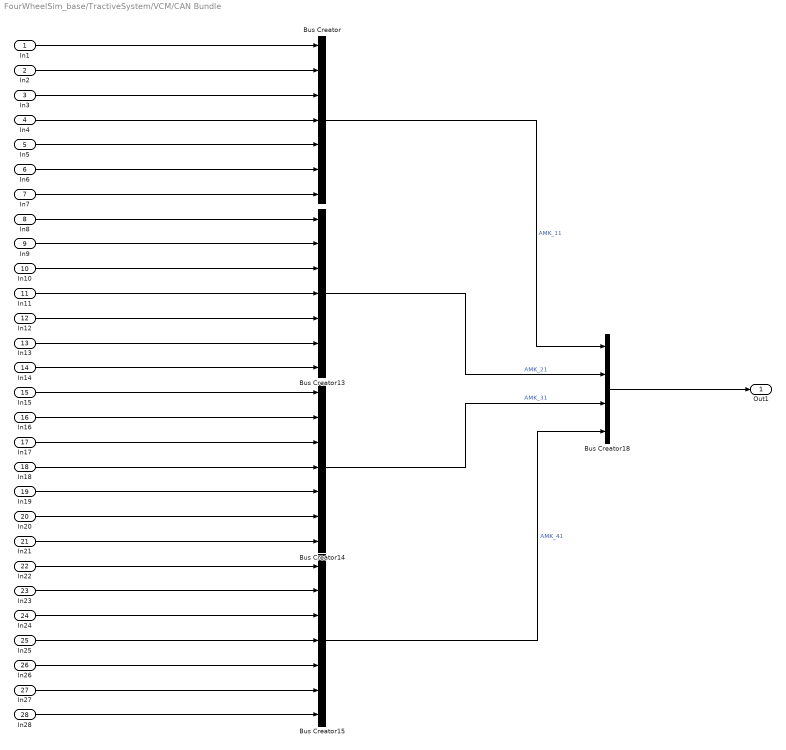
== system FourWheelSim_base/TractiveSystem/VCM/CAN Bundle ==
  In1 : Inport
  In2 : Inport  Port=2
  In3 : Inport  Port=3
  In4 : Inport  Port=4
  In5 : Inport  Port=5
  In6 : Inport  Port=6
  In7 : Inport  Port=7
  In8 : Inport  Port=8
  In9 : Inport  Port=9
  In10 : Inport  Port=10
  In11 : Inport  Port=11
  In12 : Inport  Port=12
  In13 : Inport  Port=13
  In14 : Inport  Port=14
  In15 : Inport  Port=15
  In16 : Inport  Port=16
  In17 : Inport  Port=17
  In18 : Inport  Port=18
  In19 : Inport  Port=19
  In20 : Inport  Port=20
  In21 : Inport  Port=21
  In22 : Inport  Port=22
  In23 : Inport  Port=23
  In24 : Inport  Port=24
  In25 : Inport  Port=25
  In26 : Inport  Port=26
  In27 : Inport  Port=27
  In28 : Inport  Port=28
  Bus Creator{,13..15} (4 alike) : BusCreator  Inputs=7
  Bus Creator18 : BusCreator  Inputs=4
  Out1 : Outport  VectorParamsAs1DForOutWhenUnconnected=off
  wires:
  In7/1 -> Bus Creator/7
  In6/1 -> Bus Creator/6
  In5/1 -> Bus Creator/5
  In4/1 -> Bus Creator/4
  In3/1 -> Bus Creator/3
  In2/1 -> Bus Creator/2
  In1/1 -> Bus Creator/1
  Bus Creator18/1 -> Out1/1
  In8/1 -> Bus Creator13/1
  In18/1 -> Bus Creator14/4
  In13/1 -> Bus Creator13/6
  In28/1 -> Bus Creator15/7
  Bus Creator14/1 -> Bus Creator18/3  "AMK_31"
  In19/1 -> Bus Creator14/5
  In22/1 -> Bus Creator15/1
  In11/1 -> Bus Creator13/4
  Bus Creator/1 -> Bus Creator18/1  "AMK_11"
  In26/1 -> Bus Creator15/5
  In27/1 -> Bus Creator15/6
  In23/1 -> Bus Creator15/2
  In14/1 -> Bus Creator13/7
  In21/1 -> Bus Creator14/7
  Bus Creator15/1 -> Bus Creator18/4  "AMK_41"
  In17/1 -> Bus Creator14/3
  In25/1 -> Bus Creator15/4
  Bus Creator13/1 -> Bus Creator18/2  "AMK_21"
  In20/1 -> Bus Creator14/6
  In15/1 -> Bus Creator14/1
  In9/1 -> Bus Creator13/2
  In10/1 -> Bus Creator13/3
  In24/1 -> Bus Creator15/3
  In16/1 -> Bus Creator14/2
  In12/1 -> Bus Creator13/5

== system FourWheelSim_base/TractiveSystem/VCM/speedlimit ==
  rpm : Inport
  kph : Inport  Port=2
  Min : MinMax  Inputs=2
  kph to motor rpm : Subsystem
  speedlimit(rpm) : Outport  VectorParamsAs1DForOutWhenUnconnected=off
  wires:
  kph to motor rpm/1(rpm) -> Min/2
  rpm/1 -> Min/1
  Min/1 -> speedlimit(rpm)/1
  kph/1 -> kph to motor rpm/1(kph)

== system FourWheelSim_base/4-wheel Vehicle model/comb slip model/Load/RL Load Diff ==
  note: VD講座第9回参照
  note: 横加速度による荷重移動
  FrontLoad : Inport
  RearLoad : Inport  Port=2
  LatG : Inport  Port=3
  Front Load Diff : Gain  Gain=M/df*(krfr*(hg-rch)+(1-WBf)*rcf)
  Gain : Gain  Gain=-1
  Gain1 : Gain  Gain=-1
  Rear_Load Diff1 : Gain  Gain=M/dr*((1-krfr)*(hg-rch)+WBf*rcr)
  Saturation Dynamic : simulink/Discontinuities/Saturation Dynamic  OutMin=[]  OutMax=[]  OutDataTypeStr=Inherit: Same as second input  OutDataType=fixdt(1, 16)  OutScaling=2^-10  DoSatur=off
  Saturation Dynamic2 : simulink/Discontinuities/Saturation Dynamic  OutMin=[]  OutMax=[]  OutDataTypeStr=Inherit: Same as second input  OutDataType=fixdt(1, 16)  OutScaling=2^-10  DoSatur=off
  Front Load Diff_RL : Outport  VectorParamsAs1DForOutWhenUnconnected=off
  Rear Load Diff_RL : Outport  Port=2  VectorParamsAs1DForOutWhenUnconnected=off
  wires:
  Gain1/1 -> Saturation Dynamic2/3
  Saturation Dynamic/1 -> Front Load Diff_RL/1
  LatG/1 -> Front Load Diff/1, Rear_Load Diff1/1
  RearLoad/1 -> Saturation Dynamic2/1, Gain1/1
  Rear_Load Diff1/1 -> Saturation Dynamic2/2
  FrontLoad/1 -> Gain/1, Saturation Dynamic/1
  Gain/1 -> Saturation Dynamic/3
  Front Load Diff/1 -> Saturation Dynamic/2
  Saturation Dynamic2/1 -> Rear Load Diff_RL/1
